simulink model "cartpole_simulink"  (R2020b)
settings: Solver=FixedStepAuto  StartTime=0.0  StopTime=10  FixedStep=1e-3  MaxStep=1e-3  RelTol=1e-3
model workspace (MAT data in the model file):
  g = Simulink.Parameter
  g.Value = 9.80665
  g.Description = 'gravity on earth'
  g.DataType = 'auto'
  g.DocUnits = 'm/s/s'
  g.Dimensions = [1 1]
  length_pole = Simulink.Parameter
  length_pole.Value = 0.5
  length_pole.Description = 'length of the pole/pendulum'
  length_pole.DataType = 'auto'
  length_pole.Min = 0
  length_pole.DocUnits = 'm'
  length_pole.Dimensions = [1 1]
  mass_cart = Simulink.Parameter
  mass_cart.Value = 1
  mass_cart.Description = 'mass of the cart'
  mass_cart.DataType = 'auto'
  mass_cart.Min = 0
  mass_cart.DocUnits = 'kg'
  mass_cart.Dimensions = [1 1]
  mass_pole = Simulink.Parameter
  mass_pole.Value = 0.1
  mass_pole.Description = 'mass of the pole'
  mass_pole.DataType = 'auto'
  mass_pole.Min = 0
  mass_pole.DocUnits = 'kg'
  mass_pole.Dimensions = [1 1]
  theta_0 = Simulink.Parameter
  theta_0.Value = Simulink.data.Expression
  theta_0.Value.ExpressionString = "24*rand(1)-12"
  theta_0.Description = 'starting angle of the pole'
  theta_0.DataType = 'auto'
  theta_0.DocUnits = 'deg'
  theta_0.Dimensions = -1
  x_0 = Simulink.Parameter
  x_0.Value = 0
  x_0.Description = 'starting position of the cart'
  x_0.DataType = 'auto'
  x_0.Min = -1
  x_0.Max = 1
  x_0.DocUnits = 'm'
  x_0.Dimensions = [1 1]
libraries: simulink_gym x2
settings Model: OrderedModelArguments=off  Creator=johannes  LastModifiedBy=jbrust
settings DataIOCC: ReturnWorkspaceOutputs=off  SignalLoggingName=logsoutSimulink
settings DebuggingCC: AlgebraicLoopMsg=none  ArithmeticOperatorsInVariantConditions=warning
settings SFSimCC: CustomCodeUndefinedFunction=UseInterfaceOnly

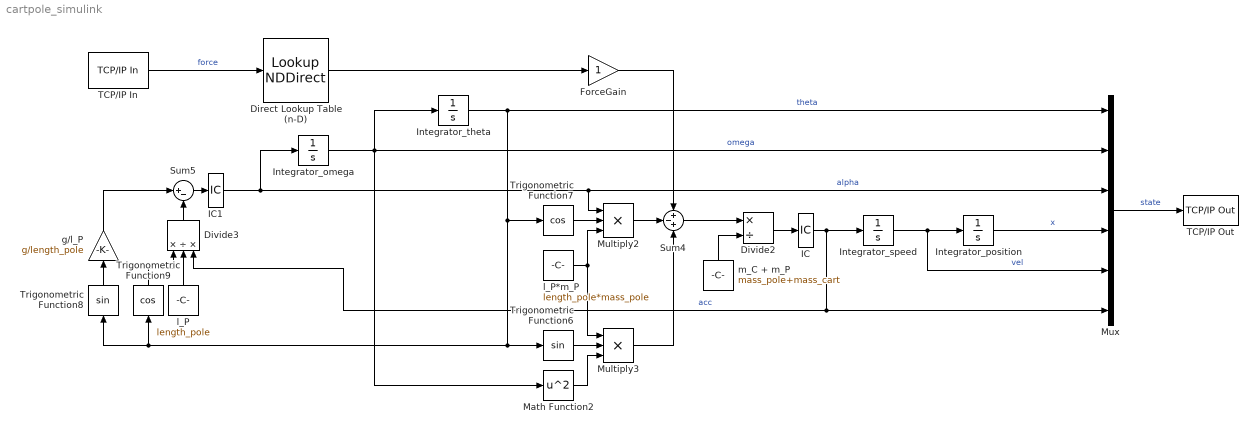
== system cartpole_simulink ==
  Direct Lookup Table (n-D) : LookupNDDirect  NumberOfTableDimensions=1  Table=[-1 0 1]  DiagnosticForOutOfRangeInput=Error
  Divide2 : Product  Inputs=*/
  Divide3 : Product  Inputs=*/*
  ForceGain : Gain
  IC : InitialCondition  Value=0
  IC1 : InitialCondition  Value=0
  Integrator_omega : Integrator
  Integrator_position : Integrator  InitialCondition=x_0  LimitOutput=on  UpperSaturationLimit=1  LowerSaturationLimit=-1
  Integrator_speed : Integrator
  Integrator_theta : Integrator  InitialCondition=theta_0*pi/180
  Math Function2 : Math  Operator=square  SignedPower=on  SaturateOnIntegerOverflow=on
  Multiply2 : Product  Inputs=3
  Multiply3 : Product  Inputs=3
  Mux : Mux  Inputs=6
  Sum4 : Sum  Inputs=+-+
  Sum5 : Sum  Inputs=|+-
  TCP/IP In : simulink_gym/TCP//IP In  port=42313  num_signals=1  t_s=1e-1
      settings: SourceProductName=Simulink Gym
  TCP/IP Out : simulink_gym/TCP//IP Out  port=42312  t_s=1e-1
      settings: SourceProductName=Simulink Gym
  Trigonometric Function6 : Trigonometry
  Trigonometric Function7 : Trigonometry  Operator=cos
  Trigonometric Function8 : Trigonometry
  Trigonometric Function9 : Trigonometry  Operator=cos
  g/l_P : Gain  Gain=g/length_pole
  l_P : Constant  Value=length_pole
  l_P*m_P : Constant  Value=length_pole*mass_pole
  m_C + m_P : Constant  Value=mass_pole+mass_cart
  wires:
  Divide2/1 -> IC/1
  Integrator_speed/1 -> Mux/5, Integrator_position/1  "vel"
  Integrator_omega/1 -> Mux/2, Math Function2/1, Integrator_theta/1  "omega"
  Trigonometric Function7/1 -> Multiply2/2
  Integrator_theta/1 -> Mux/1, Trigonometric Function7/1, Trigonometric Function6/1, Trigonometric Function9/1, Trigonometric Function8/1  "theta"
  Integrator_position/1 -> Mux/4  "x"
  Sum5/1 -> IC1/1
  m_C + m_P/1 -> Divide2/2
  Multiply2/1 -> Sum4/2
  l_P*m_P/1 -> Multiply3/1, Multiply2/3
  Multiply3/1 -> Sum4/3
  Math Function2/1 -> Multiply3/3
  Trigonometric Function6/1 -> Multiply3/2
  g/l_P/1 -> Sum5/1
  Trigonometric Function8/1 -> g/l_P/1
  Trigonometric Function9/1 -> Divide3/1
  Divide3/1 -> Sum5/2
  l_P/1 -> Divide3/2
  IC/1 -> Mux/6, Divide3/3, Integrator_speed/1  "acc"
  IC1/1 -> Integrator_omega/1, Mux/3, Multiply2/1  "alpha"
  Sum4/1 -> Divide2/1
  Mux/1 -> TCP/IP Out/1  "state"
  TCP/IP In/1 -> Direct Lookup Table (n-D)/1  "force"
  ForceGain/1 -> Sum4/1
  Direct Lookup Table (n-D)/1 -> ForceGain/1
